simulink model "simulate_complexBaseband_PM_FM"  (R2017a)
settings: Solver=VariableStepAuto  StartTime=0.0  StopTime=1  RelTol=1e-3
InitFcn:
  | fs = 1e4;
  | frameSize = 1000;
undefined symbols (not defined in the file): DiscIntNeverNeededParam
libraries: dspsrcs4 x4, simulink x1
settings Model: Creator=prust  LastModifiedBy=prust

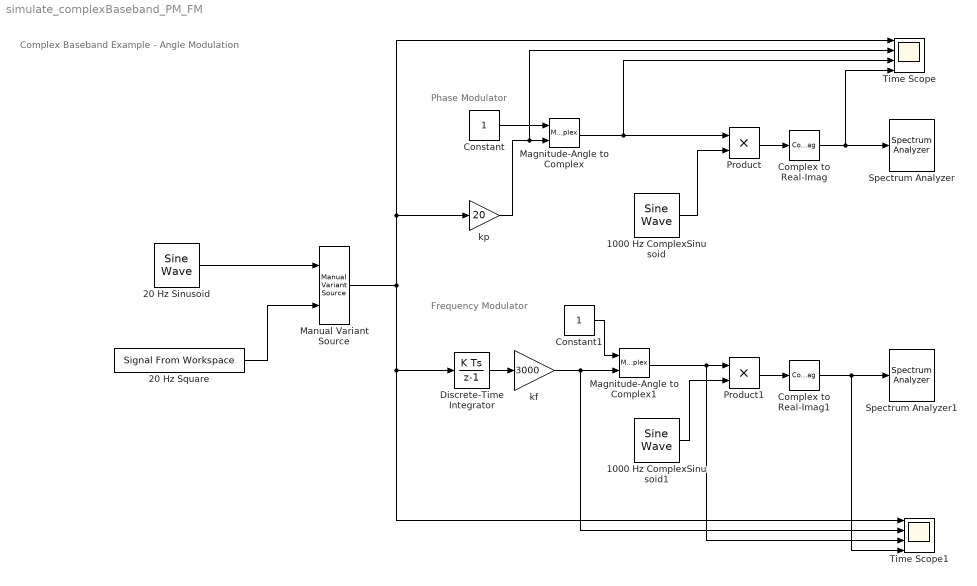
== system simulate_complexBaseband_PM_FM ==
  note: Frequency Modulator
  note: Phase Modulator
  note: Complex Baseband Example - Angle Modulation
  1000 Hz ComplexSinusoid : dspsrcs4/Sine Wave  Amplitude=sqrt(2)  Frequency=1000  Phase=0  SampleMode=Discrete  OutComplex=Complex  CompMethod=Trigonometric fcn  TableSize=Speed  SampleTime=1/fs  SamplesPerFrame=1  ResetState=Restart at time zero  OutputFrames=off  dataType=double  wordLen=16  udDataType=sfix(16)  fracBitsMode=Best precision  numFracBits=15  OutDataTypeStr=double  LastOutDataTypeStr=double
  1000 Hz ComplexSinusoid1 : dspsrcs4/Sine Wave  Amplitude=sqrt(2)  Frequency=1000  Phase=0  SampleMode=Discrete  OutComplex=Complex  CompMethod=Trigonometric fcn  TableSize=Speed  SampleTime=1/fs  SamplesPerFrame=1  ResetState=Restart at time zero  OutputFrames=off  dataType=double  wordLen=16  udDataType=sfix(16)  fracBitsMode=Best precision  numFracBits=15  OutDataTypeStr=double  LastOutDataTypeStr=double
  20 Hz Sinusoid : dspsrcs4/Sine Wave  Amplitude=1  Frequency=20  Phase=0  SampleMode=Discrete  OutComplex=Real  CompMethod=Trigonometric fcn  TableSize=Speed  SampleTime=1/fs  SamplesPerFrame=1  ResetState=Restart at time zero  OutputFrames=off  dataType=double  wordLen=16  udDataType=sfix(16)  fracBitsMode=Best precision  numFracBits=15  OutDataTypeStr=double  LastOutDataTypeStr=double
  20 Hz Square : dspsrcs4/Signal From Workspace  X=[ones(250,1); -ones(250,1)]  Ts=1/fs  nsamps=1  OutputAfterFinalValue=Cyclic repetition  ignoreOrWarnInputAndFrameLengths=off  OutputFrames=off
  Complex to Real-Imag : ComplexToRealImag  Output=Real
  Complex to Real-Imag1 : ComplexToRealImag  Output=Real
  Constant : Constant
  Constant1 : Constant
  Discrete-Time Integrator : DiscreteIntegrator  InitialConditionSetting=State (most efficient)  SampleTime=-1  ICPrevOutput=DiscIntNeverNeededParam  ICPrevScaledInput=DiscIntNeverNeededParam
  Magnitude-Angle to Complex : MagnitudeAngleToComplex
  Magnitude-Angle to Complex1 : MagnitudeAngleToComplex
  Manual Variant Source : simulink/Signal Routing/Manual Variant Source  NumChoices=2  OverrideUsingVariant=V_2
      settings: SourceProductName=Simulink
  Product : Product
  Product1 : Product
  Spectrum Analyzer : SpectrumAnalyzer
  Spectrum Analyzer1 : SpectrumAnalyzer
  Time Scope : Scope  NumInputPorts=4
  Time Scope1 : Scope  NumInputPorts=4
  kf : Gain  Gain=3000
  kp : Gain  Gain=20
  wires:
  Constant/1 -> Magnitude-Angle to Complex/1
  Magnitude-Angle to Complex/1 -> Time Scope/3, Product/1
  1000 Hz ComplexSinusoid/1 -> Product/2
  Product/1 -> Complex to Real-Imag/1
  Complex to Real-Imag/1 -> Time Scope/4, Spectrum Analyzer/1
  kp/1 -> Time Scope/2, Magnitude-Angle to Complex/2
  Discrete-Time Integrator/1 -> kf/1
  kf/1 -> Magnitude-Angle to Complex1/2, Time Scope1/2
  Manual Variant Source/1 -> kp/1, Time Scope/1, Discrete-Time Integrator/1, Time Scope1/1
  1000 Hz ComplexSinusoid1/1 -> Product1/2
  Complex to Real-Imag1/1 -> Spectrum Analyzer1/1, Time Scope1/4
  Product1/1 -> Complex to Real-Imag1/1
  Magnitude-Angle to Complex1/1 -> Time Scope1/3, Product1/1
  Constant1/1 -> Magnitude-Angle to Complex1/1
  20 Hz Sinusoid/1 -> Manual Variant Source/1
  20 Hz Square/1 -> Manual Variant Source/2
